simulink model "missile"  (R2026a)
settings: Solver=ode4  StopTime=T_MAX  FixedStep=CODEGEN_STEP
PreLoadFcn:
  | run(fullfile(fileparts(which('missile')), 'model', 'missile_params.m'));
undefined symbols (not defined in the file): R_M0, V_M_INIT
settings Model: Creator=jerem  LastModifiedBy=jerem
settings RTWCC: SystemTargetFile=ert.tlc  Description=Embedded Coder
settings ERTTargetCC: GenerateSampleERTMain=on  CodeInterfacePackaging=Reusable function  SupportContinuousTime=on  GenerateAllocFcn=on

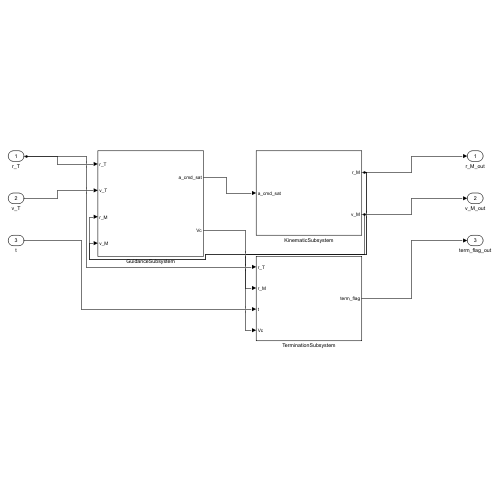
[thumbnail: Simulink's stored preview of the top-level diagram]
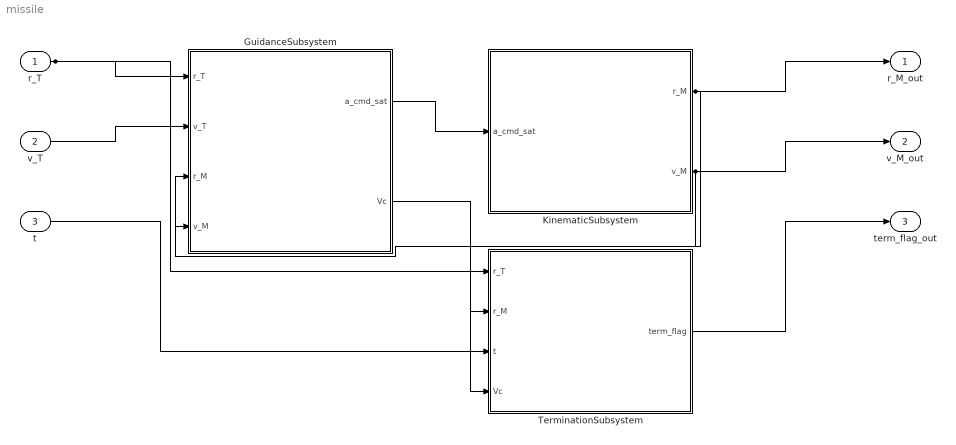
== system missile ==
  r_T : Inport  PortDimensions=3
  v_T : Inport  Port=2  PortDimensions=3
  t : Inport  Port=3  PortDimensions=1
  GuidanceSubsystem : Subsystem
  KinematicSubsystem : Subsystem
  TerminationSubsystem : Subsystem
  r_M_out : Outport
  v_M_out : Outport  Port=2
  term_flag_out : Outport  Port=3
  wires:
  r_T/1 -> GuidanceSubsystem/1(r_T), TerminationSubsystem/1(r_T)
  v_T/1 -> GuidanceSubsystem/2(v_T)
  GuidanceSubsystem/1(a_cmd_sat) -> KinematicSubsystem/1(a_cmd_sat)
  KinematicSubsystem/1(r_M) -> GuidanceSubsystem/3(r_M), r_M_out/1, TerminationSubsystem/2(r_M)
  KinematicSubsystem/2(v_M) -> GuidanceSubsystem/4(v_M), v_M_out/1
  t/1 -> TerminationSubsystem/3(t)
  GuidanceSubsystem/2(Vc) -> TerminationSubsystem/4(Vc)
  TerminationSubsystem/1(term_flag) -> term_flag_out/1

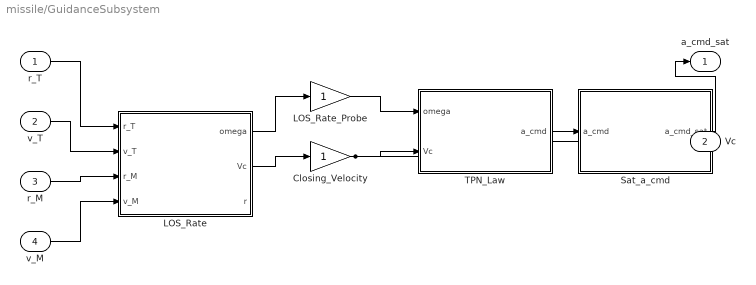
== system missile/GuidanceSubsystem ==
  r_T : Inport  PortDimensions=3
  v_T : Inport  Port=2  PortDimensions=3
  r_M : Inport  Port=3  PortDimensions=3
  v_M : Inport  Port=4  PortDimensions=3
  Closing_Velocity : Gain
  LOS_Rate : MATLAB Function  TreatAsAtomicUnit=on
  LOS_Rate_Probe : Gain
  Sat_a_cmd : MATLAB Function  TreatAsAtomicUnit=on
  TPN_Law : MATLAB Function  TreatAsAtomicUnit=on
  a_cmd_sat : Outport
  Vc : Outport  Port=2
  wires:
  r_T/1 -> LOS_Rate/1(r_T)
  v_T/1 -> LOS_Rate/2(v_T)
  r_M/1 -> LOS_Rate/3(r_M)
  v_M/1 -> LOS_Rate/4(v_M)
  LOS_Rate/1(omega) -> LOS_Rate_Probe/1
  LOS_Rate/2(Vc) -> Closing_Velocity/1
  LOS_Rate_Probe/1 -> TPN_Law/1(omega)
  Closing_Velocity/1 -> TPN_Law/2(Vc), Vc/1
  TPN_Law/1(a_cmd) -> Sat_a_cmd/1(a_cmd)
  Sat_a_cmd/1(a_cmd_sat) -> a_cmd_sat/1

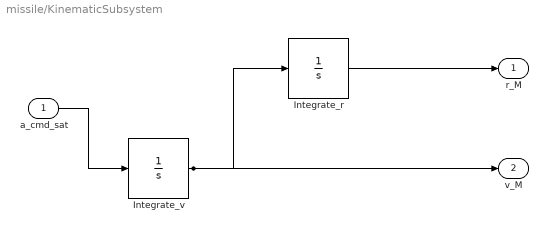
== system missile/KinematicSubsystem ==
  a_cmd_sat : Inport  PortDimensions=3
  Integrate_r : Integrator  InitialCondition=R_M0
  Integrate_v : Integrator  InitialCondition=V_M_INIT
  r_M : Outport
  v_M : Outport  Port=2
  wires:
  a_cmd_sat/1 -> Integrate_v/1
  Integrate_v/1 -> Integrate_r/1, v_M/1
  Integrate_r/1 -> r_M/1

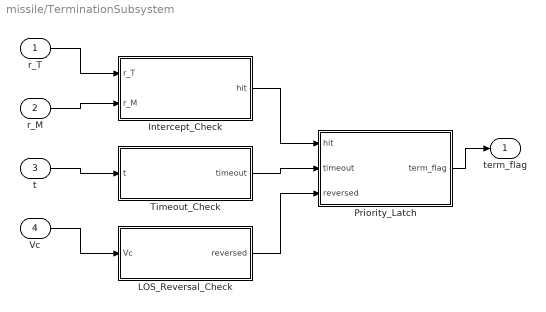
== system missile/TerminationSubsystem ==
  r_T : Inport  PortDimensions=3
  r_M : Inport  Port=2  PortDimensions=3
  t : Inport  Port=3  PortDimensions=1
  Vc : Inport  Port=4  PortDimensions=1
  Intercept_Check : MATLAB Function  TreatAsAtomicUnit=on
  LOS_Reversal_Check : MATLAB Function  TreatAsAtomicUnit=on
  Priority_Latch : MATLAB Function  TreatAsAtomicUnit=on
  Timeout_Check : MATLAB Function  TreatAsAtomicUnit=on
  term_flag : Outport
  wires:
  r_T/1 -> Intercept_Check/1(r_T)
  r_M/1 -> Intercept_Check/2(r_M)
  t/1 -> Timeout_Check/1(t)
  Vc/1 -> LOS_Reversal_Check/1(Vc)
  Intercept_Check/1(hit) -> Priority_Latch/1(hit)
  Timeout_Check/1(timeout) -> Priority_Latch/2(timeout)
  LOS_Reversal_Check/1(reversed) -> Priority_Latch/3(reversed)
  Priority_Latch/1(term_flag) -> term_flag/1

== matlab function missile/GuidanceSubsystem/TPN_Law ==
  data: omega input; a_cmd output; Vc input
function a_cmd = fcn(omega, Vc)
%#codegen
    N = 4;              % baked in at build time from missile_params.m
    a_cmd = N * Vc * omega;
end

== matlab function missile/GuidanceSubsystem/LOS_Rate ==
  data: r_T input; omega output; v_T input; r_M input; v_M input; Vc output; r output
function [omega, Vc, r] = fcn(r_T, v_T, r_M, v_M)
%#codegen
    r     = r_T - r_M;               % relative position
    r_dot = v_T - v_M;               % relative velocity
    r_mag = norm(r);
    if r_mag < 1e-6
        omega = zeros(3,1);
        Vc    = 0;
    else
        omega = cross(r, r_dot) / (r_mag*r_mag);
        Vc    = -dot(r, r_dot) / r_mag;
    end
end

== matlab function missile/GuidanceSubsystem/Sat_a_cmd ==
  data: a_cmd input; a_cmd_sat output
function a_cmd_sat = fcn(a_cmd)
%#codegen
    LATAX_MAX = 392.4;   % baked in at build time from missile_params.m
    mag = norm(a_cmd);
    if mag > LATAX_MAX
        a_cmd_sat = a_cmd * (LATAX_MAX / mag);
    else
        a_cmd_sat = a_cmd;
    end
end

== matlab function missile/TerminationSubsystem/Intercept_Check ==
  data: r_T input; hit output; r_M input
function hit = fcn(r_T, r_M)
%#codegen
    R_LETHAL = 25;   % baked in at build time from missile_params.m
    hit = double(norm(r_T - r_M) < R_LETHAL);
end

== matlab function missile/TerminationSubsystem/Timeout_Check ==
  data: t input; timeout output
function timeout = fcn(t)
%#codegen
    T_MAX = 60;   % baked in at build time from missile_params.m
    timeout = double(t >= T_MAX);
end

== matlab function missile/TerminationSubsystem/LOS_Reversal_Check ==
  settings: updateMethod=DISCRETE  sampleTime=CODEGEN_STEP
  data: Vc input; reversed output
function reversed = fcn(Vc)
%#codegen
    persistent Vc_peak
    if isempty(Vc_peak)
        Vc_peak = -inf;
    end
    if Vc > Vc_peak
        Vc_peak = Vc;
    end
    reversed = double((Vc_peak > 0) && (Vc < 0));
end

== matlab function missile/TerminationSubsystem/Priority_Latch ==
  settings: updateMethod=DISCRETE  sampleTime=CODEGEN_STEP
  data: hit input; term_flag output; timeout input; reversed input
function term_flag = fcn(hit, timeout, reversed)
%#codegen
    persistent latched
    if isempty(latched)
        latched = int32(0);
    end
    if latched == 0
        if hit ~= 0
            latched = int32(1);
        elseif timeout ~= 0
            latched = int32(2);
        elseif reversed ~= 0
            latched = int32(3);
        end
    end
    term_flag = double(latched);
end
